simulink model "mpc_pendcartImplicitMPC"  (R2024b)
settings: Solver=ode15s  StartTime=0.0  StopTime=30  MaxStep=1e-3  RelTol=1e-3  EnableMultiTasking=on
libraries: SignalEditorBlockLib x1, mpclib x1
settings Model: Creator=The MathWorks, Inc.
settings SolverCC: AlgebraicLoopSolver=LineSearch  MinimalZcImpactIntegration=on
settings DataIOCC: LimitDataPoints=on  SaveFormat=Array  ReturnWorkspaceOutputs=off
settings OptimizationCC: ReuseModelBlockBuffer=off  LifeSpan=inf
settings DebuggingCC: AlgebraicLoopMsg=none  UnderspecifiedInitializationDetection=Classic  MergeDetectMultiDrivingBlocksExec=none  SolverPrmCheckMsg=warning  UnconnectedInputMsg=warning  UnconnectedOutputMsg=warning  UnconnectedLineMsg=warning  AllowSymbolicDim=off  StateNameClashWarn=warning  SubsystemReferenceDiagnosticForUnitTest=warning  SFUnexpectedBacktrackingDiag=warning  SFNoUnconditionalDefaultTransitionDiag=warning  SFExecutionAtInitializationDiag=none  ArithmeticOperatorsInVariantConditions=warning
settings HardwareCC: ProdBitPerPointer=32  ProdBitPerSizeT=32  ProdBitPerPtrDiffT=32  ProdLargestAtomicFloat=None  ProdIntDivRoundTo=Undefined  ProdEndianess=Unspecified  ProdWordSize=32  ProdHWDeviceType=32-bit Generic
settings ModelReferenceCC: EnableRefExpFcnMdlSchedulingChecks=on  PropagateSignalLabelsOutOfModel=off
settings SFSimCC: SimUseLocalCustomCode=off  CustomCodeUndefinedFunction=UseInterfaceOnly
settings RTWCC: RTWUseLocalCustomCode=off  GPUComputeCapability=3.5
settings CodeAppCC: StateflowObjectComments=on
settings GRTTargetCC: TargetLangStandard=C89/C90 (ANSI)
settings ConfigComp: CovMetricSettings=dw  CovSaveCumulativeToWorkspaceVar=on  CovSaveSingleToWorkspaceVar=on  CovExternalEMLEnable=off  CovSFcnEnable=off  CovBoundaryAbsTol=1.0e-5
settings SimscapeCC: SimscapeNormalizeSystem=off
settings ConfigurationSet: Description=SimMechanics 2G
settings ExplorerConfigSet: InternalSimMechanicsExplorerSettings="<ExplorerConfiguration><canonicalview>default</canonicalview><AnimationSetting><BasePlaybackSpeed>1.0</BasePlaybackSpeed><PlaybackSpeedFactor>1.0</PlaybackSpeedFactor></AnimationSetting><TilePanel><TileInfo><Tiles Columns=\"1\" Count=\"1\" Rows=\"1\"><Column Left=\"2\" Weight=\"1\"/><Column Left=\"1552\"/><Row Top=\"2\" Weight=\"1\"/><Row Top=\"932\"/><Tile Height=\"1\" Width=\"1\" X=\"0\" Y=\"0\"/></Tiles></TileInfo><SceneInfo><SceneViewer><BGColor><R>0.60000002384185791</R><G>0.60000002384185791</G><B>0.60000002384185791</B></BGColor><Camera><Position><X>0.027865189060748197</X><Y>-2.5719092456962986</Y><Z>0.23157896538506753</Z></Position><Center><X>0.62659712312732463</X><Y>-0.46110119691712204</Y><Z>0.22087365386473376</Z></Center><Up><X>-0.0079438354874226333</X><Y>0.0073246425924307582</Y><Z>0.99994162084025784</Z></Up><Left>-0.24533778208815546</Left><Right>0.24533778208815546</Right><Bottom>-0.79734779727023208</Bottom><Top>0.79734779727023208</Top></Camera></SceneViewer></SceneInfo></TilePanel></ExplorerConfiguration>"

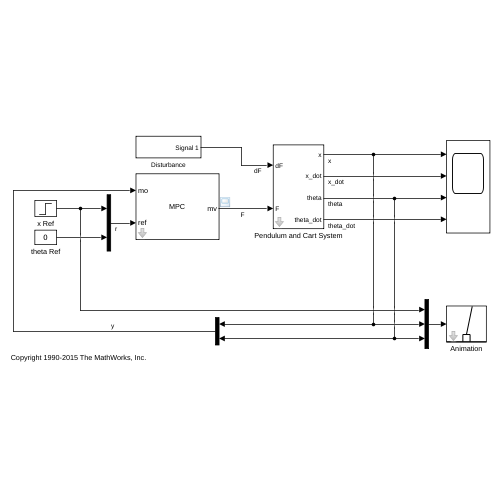
[thumbnail: Simulink's stored preview of the top-level diagram]
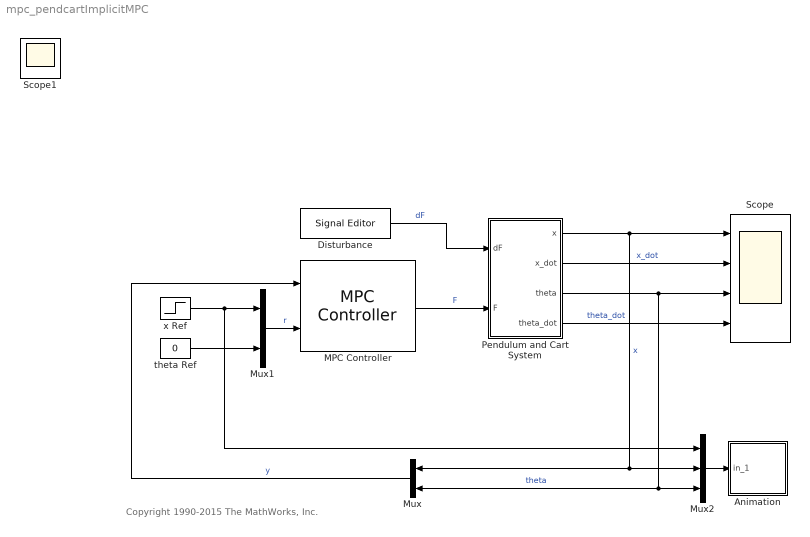
== system mpc_pendcartImplicitMPC ==
  note: Copyright 1990-2015 The MathWorks, Inc.
  Animation : Subsystem  mask(Pendulum plot){RefBlock=x Ref}
      mask prompts: RefBlock "Cart Reference Signal Block Name:"
      mask help: Pendulum plot
      mask Help: Pendulum animation function using Handle graphics.
      mask Display: plot([-10 10],[0 0],[-2 -2 2 2],[0 1 1 0],[0 3],[1 5])
  Disturbance : SignalEditorBlockLib/Signal Editor  FileName=pendulumDisturbanceLTI.mat  ActiveScenario=Group_1  ActiveSignal=Signal 1  IsBus=off  OutputBusObjectStr=Bus: BusObject  SampleTime=0  OutputAfterFinalValue=Extrapolation  Unit=inherit  PreserveSignalName=on  ApplySigPropsToAllScenarios=on  ApplySigPropsToAllSignals=off
  MPC Controller : mpclib/MPC Controller  mpcobj=mpcobj  x0=[]  is_multiple=0  enable_value=0  return_u0=off  updateMPCinCallerWorkspace=on  md_inport=off  mv_inport=off  uref_inport=off  return_cost=off  return_mvseq=off  return_qpstatus=off  return_xseq=off  return_state=off  return_ovseq=off  state_inport=off  umin_inport=off  umax_inport=off  ymin_inport=off  ymax_inport=off  cc_inport=off  ywt_inport=off  uwt_inport=off  duwt_inport=off  rhoeps_inport=off  pm_inport=off  MaximumP=10  HorizonChoice=FixedHorizon  n_ts=0.01  n_p=50  n_mv=1  n_md=0  n_ud=1  n_mo=2  n_uo=0  BlockDataType=double  SampleTimeInherited=off  switch_inport=off
  Mux : Mux  Inputs=2
  Mux1 : Mux  Inputs=2
  Mux2 : Mux  Inputs=3
  Pendulum and Cart System : Subsystem  mask{MCart=1, m=1, g=9.81, l=0.5, Kd=10, x0=0, theta0=0}
      mask prompts: MCart "Cart mass (Kg)"; m "Pendulum mass (Kg)"; g "Gravity (m/s^2)"; l "Distance from joint to pendulum center of mass (m)"; Kd "Viscous friction coefficient on cart (N*s/m)"; x0 "Initial cart position (m)"; theta0 "Initial pendulum angle (rad)"
      mask help:
      | Pendulum and Cart System
      |
      | The block represents a pendulum attached to an unactuated revolutionary joint on a cart, which moves along a one-dimensional track subject to viscous damping.
      |
      | The block inputs are the force F on the cart and the force dF on the pendulum. The block outputs are the four system states: linear position and velocity or the cart (rightward-positive), angular position and velocity of the pendulum (counterclockwise-positive, with the upright position being zero radians).
      |
      | Look under the mask to see the equations and their Simulink implementation. For a derivation of the system equations, click Help.
      mask Help: web('https://www.mathworks.com/help/symbolic/derive-and-simulate-cart-pole-system.html')
  Scope : Scope  NumInputPorts=4
  theta Ref : Constant  Value=0
  x Ref : Step  After=10  SampleTime=0
  Scope1 : Scope
  wires:
  theta Ref/1 -> Mux1/2
  Mux/1 -> MPC Controller/1  "y"
  Pendulum and Cart System/4(theta_dot) -> Scope/4  "theta_dot"
  Pendulum and Cart System/3(theta) -> Mux/2, Mux2/3, Scope/3  "theta"
  Pendulum and Cart System/2(x_dot) -> Scope/2  "x_dot"
  Pendulum and Cart System/1(x) -> Mux/1, Mux2/2, Scope/1  "x"
  Disturbance/1 -> Pendulum and Cart System/1(dF)  "dF"
  Mux1/1 -> MPC Controller/2  "r"
  MPC Controller/1 -> Pendulum and Cart System/2(F)  "F"
  Mux2/1 -> Animation/1(in_1)
  x Ref/1 -> Mux2/1, Mux1/1

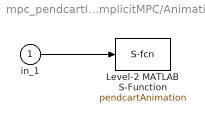
== system mpc_pendcartImplicitMPC/Animation ==
  in_1 : Inport
  Level-2 MATLAB S-Function : M-S-Function  FunctionName=pendcartAnimation  Parameters=RefBlock
  wires:
  in_1/1 -> Level-2 MATLAB S-Function/1

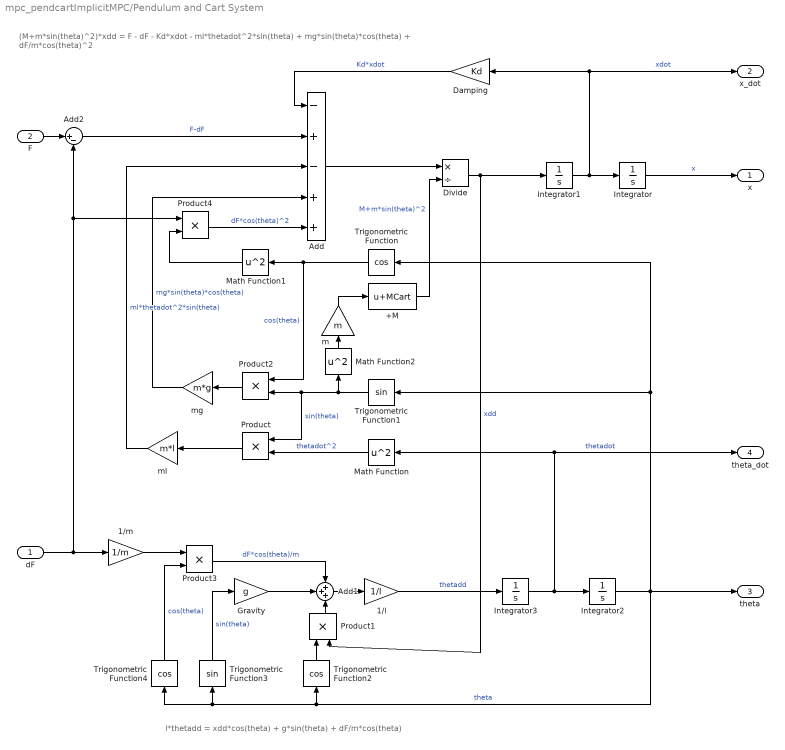
== system mpc_pendcartImplicitMPC/Pendulum and Cart System ==
  note: l*thetadd = xdd*cos(theta) + g*sin(theta) + dF/m*cos(theta)
  note: (M+m*sin(theta)^2)*xdd = F - dF - Kd*xdot - ml*thetadot^2*sin(theta) + mg*sin(theta)*cos(theta) + dF/m*cos(theta)^2
  dF : Inport
  F : Inport  Port=2
  +M : Bias  Bias=MCart  SaturateOnIntegerOverflow=off
  1/l : Gain  Gain=1/l
  1/m : Gain  Gain=1/m
  Add : Sum  Inputs=-+-++
  Add1 : Sum  Inputs=+++
  Add2 : Sum  Inputs=|+-
  Damping : Gain  Gain=Kd
  Divide : Product  Inputs=*/
  Gravity : Gain  Gain=g
  Integrator : Integrator  InitialCondition=x0  ContinuousStateAttributes='x'
  Integrator1 : Integrator  ContinuousStateAttributes='xdot'
  Integrator2 : Integrator  InitialCondition=theta0  ContinuousStateAttributes='theta'
  Integrator3 : Integrator  ContinuousStateAttributes='thetadot'
  Math Function : Math  Operator=square  SignedPower=on
  Math Function1 : Math  Operator=square  SignedPower=on
  Math Function2 : Math  Operator=square  SignedPower=on
  Product{,1..4} (5 alike) : Product
  Trigonometric Function : Trigonometry  Operator=cos
  Trigonometric Function1 : Trigonometry
  Trigonometric Function2 : Trigonometry  Operator=cos
  Trigonometric Function3 : Trigonometry
  Trigonometric Function4 : Trigonometry  Operator=cos
  m : Gain  Gain=m
  mg : Gain  Gain=m*g
  ml : Gain  Gain=m*l
  x : Outport  VectorParamsAs1DForOutWhenUnconnected=off
  x_dot : Outport  Port=2  VectorParamsAs1DForOutWhenUnconnected=off
  theta : Outport  Port=3  VectorParamsAs1DForOutWhenUnconnected=off
  theta_dot : Outport  Port=4  VectorParamsAs1DForOutWhenUnconnected=off
  wires:
  Product/1 -> ml/1
  ml/1 -> Add/3  "ml*thetadot^2*sin(theta)"
  Add2/1 -> Add/2  "F-dF"
  Add1/1 -> 1/l/1
  Product2/1 -> mg/1
  Integrator1/1 -> Damping/1, x_dot/1, Integrator/1  "xdot"
  Integrator/1 -> x/1  "x"
  Trigonometric Function1/1 -> Math Function2/1, Product2/2, Product/1  "sin(theta)"
  Trigonometric Function2/1 -> Product1/1
  Divide/1 -> Integrator1/1, Product1/2  "xdd"
  Add/1 -> Divide/1
  Product3/1 -> Add1/1  "dF*cos(theta)/m"
  Integrator2/1 -> Trigonometric Function2/1, Trigonometric Function4/1, Trigonometric Function3/1, theta/1, Trigonometric Function1/1, Trigonometric Function/1  "theta"
  Integrator3/1 -> theta_dot/1, Math Function/1, Integrator2/1  "thetadot"
  Trigonometric Function/1 -> Product2/1, Math Function1/1  "cos(theta)"
  Gravity/1 -> Add1/2
  Trigonometric Function3/1 -> Gravity/1  "sin(theta)"
  F/1 -> Add2/1
  Damping/1 -> Add/1  "Kd*xdot"
  Trigonometric Function4/1 -> Product3/2  "cos(theta)"
  1/m/1 -> Product3/1
  dF/1 -> Product4/1, Add2/2, 1/m/1
  1/l/1 -> Integrator3/1  "thetadd"
  Math Function/1 -> Product/2  "thetadot^2"
  Product1/1 -> Add1/3
  mg/1 -> Add/4  "mg*sin(theta)*cos(theta)"
  Math Function1/1 -> Product4/2
  Product4/1 -> Add/5  "dF*cos(theta)^2"
  Math Function2/1 -> m/1
  +M/1 -> Divide/2  "M+m*sin(theta)^2"
  m/1 -> +M/1
